simulink model "ele"  (R2023a)
settings: Solver=VariableStepAuto  StartTime=0.0  StopTime=20  RelTol=1e-3
values from neighbouring files (symbols this model uses):
  waypointData_front = [-1.88818518125 -2.2600318378 -2.41179824016 -2.35548053674 -2.22744803538 -2.06210458742 -1.82611832354 -1.58946605338 -1.25340747671 -1.54604493893 -1.70384741821 -1.82785013395 ... (45 elements, 15x3)]    [dat.mat]
  waypointData_hind = [-1.88818518125 -1.55059762067 -1.31714165015 -1.07851127829 -0.915846032516 -0.785511813404 -0.729794322428 -0.881560682034 -1.25340747671 -1.16436080646 -1.21961717711 -1.31374250977 ... (45 elements, 15x3)]    [dat.mat]
undefined symbols (not defined in the file or in its folder): X, Y, Z
libraries: sm_lib x122, nesl_utility x62, robotmaniplib x16, robotcorelib x16
(part 1 of 4)
settings Model: Creator=mkris  LastModifiedBy=mkris

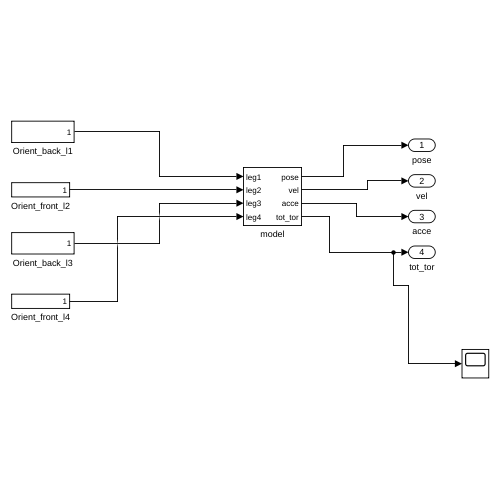
[thumbnail: Simulink's stored preview of the top-level diagram]
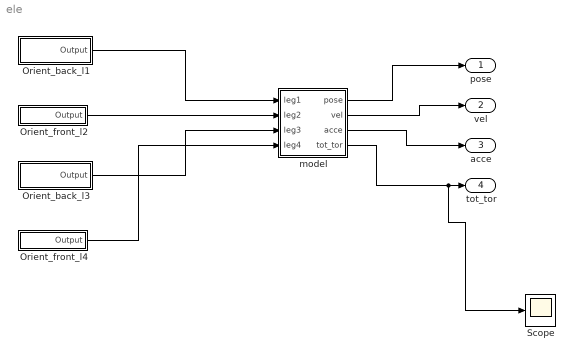
== system ele ==
  Orient_back_l1 : Subsystem
  Orient_back_l3 : Subsystem
  Orient_front_l2 : Subsystem
  Orient_front_l4 : Subsystem
  Scope : Scope
  model : Subsystem
  pose : Outport
  vel : Outport  Port=2
  acce : Outport  Port=3
  tot_tor : Outport  Port=4
  wires:
  model/1(pose) -> pose/1
  model/2(vel) -> vel/1
  model/3(acce) -> acce/1
  model/4(tot_tor) -> Scope/1, tot_tor/1
  Orient_back_l1/1(Output) -> model/1(leg1)
  Orient_front_l2/1(Output) -> model/2(leg2)
  Orient_back_l3/1(Output) -> model/3(leg3)
  Orient_front_l4/1(Output) -> model/4(leg4)

== system ele/Orient_back_l1 ==
  Clock1 : Clock
  If : If  IfExpression=u1 < 5  ElseIfExpressions=u1 < 10,u1 < 15
  Merge : Merge  Inputs=4
  down2 : Subsystem  TreatAsAtomicUnit=on
  down3 : Subsystem  TreatAsAtomicUnit=on
  down4 : Subsystem  TreatAsAtomicUnit=on
  up : Subsystem  TreatAsAtomicUnit=on
  Output : Outport
  wires:
  down4/1(Out1) -> Merge/3
  down3/1(Out1) -> Merge/4
  If/4 -> down4/Action
  If/3 -> down3/Action
  If/2 -> down2/Action
  up/1(Output) -> Merge/1
  Clock1/1 -> If/1, up/1(Input), down2/1(In1), down3/1(In1), down4/1(In1)
  down2/1(Out1) -> Merge/2
  If/1 -> up/Action
  Merge/1 -> Output/1

== system ele/Orient_back_l3 ==
  Clock1 : Clock
  If : If  IfExpression=u1 < 5  ElseIfExpressions=u1 < 10,u1 < 15
  Merge : Merge  Inputs=4
  down2 : Subsystem  TreatAsAtomicUnit=on
  down3 : Subsystem  TreatAsAtomicUnit=on
  down4 : Subsystem  TreatAsAtomicUnit=on
  up : Subsystem  TreatAsAtomicUnit=on
  Output : Outport
  wires:
  Merge/1 -> Output/1
  If/1 -> down3/Action
  down4/1(Out1) -> Merge/2
  Clock1/1 -> down2/1(In1), up/1(Input), down4/1(In1), down3/1(In1), If/1
  down3/1(Out1) -> Merge/1
  If/2 -> down4/Action
  If/3 -> up/Action
  If/4 -> down2/Action
  up/1(Output) -> Merge/4
  down2/1(Out1) -> Merge/3

== system ele/Orient_front_l2 ==
  Clock1 : Clock
  If : If  IfExpression=u1 < 5  ElseIfExpressions=u1 < 10,u1 < 15
  Merge : Merge  Inputs=4
  down2 : Subsystem  TreatAsAtomicUnit=on
  down3 : Subsystem  TreatAsAtomicUnit=on
  down4 : Subsystem  TreatAsAtomicUnit=on
  up : Subsystem  TreatAsAtomicUnit=on
  Output : Outport
  wires:
  If/1 -> down4/Action
  up/1(Output) -> Merge/2
  Clock1/1 -> down2/1(In1), down3/1(In1), up/1(Input), down4/1(In1), If/1
  down4/1(Out1) -> Merge/1
  If/2 -> up/Action
  If/3 -> down2/Action
  If/4 -> down3/Action
  down2/1(Out1) -> Merge/4
  down3/1(Out1) -> Merge/3
  Merge/1 -> Output/1

== system ele/Orient_front_l4 ==
  Clock1 : Clock
  If : If  IfExpression=u1 < 5  ElseIfExpressions=u1 < 10,u1 < 15
  Merge : Merge  Inputs=4
  down2 : Subsystem  TreatAsAtomicUnit=on
  down3 : Subsystem  TreatAsAtomicUnit=on
  down4 : Subsystem  TreatAsAtomicUnit=on
  up : Subsystem  TreatAsAtomicUnit=on
  Output : Outport
  wires:
  Merge/1 -> Output/1
  up/1(Output) -> Merge/3
  down4/1(Out1) -> Merge/4
  If/4 -> up/Action
  If/3 -> down4/Action
  If/2 -> down3/Action
  down2/1(Out1) -> Merge/1
  Clock1/1 -> down3/1(In1), down2/1(In1), If/1, down4/1(In1), up/1(Input)
  down3/1(Out1) -> Merge/2
  If/1 -> down2/Action

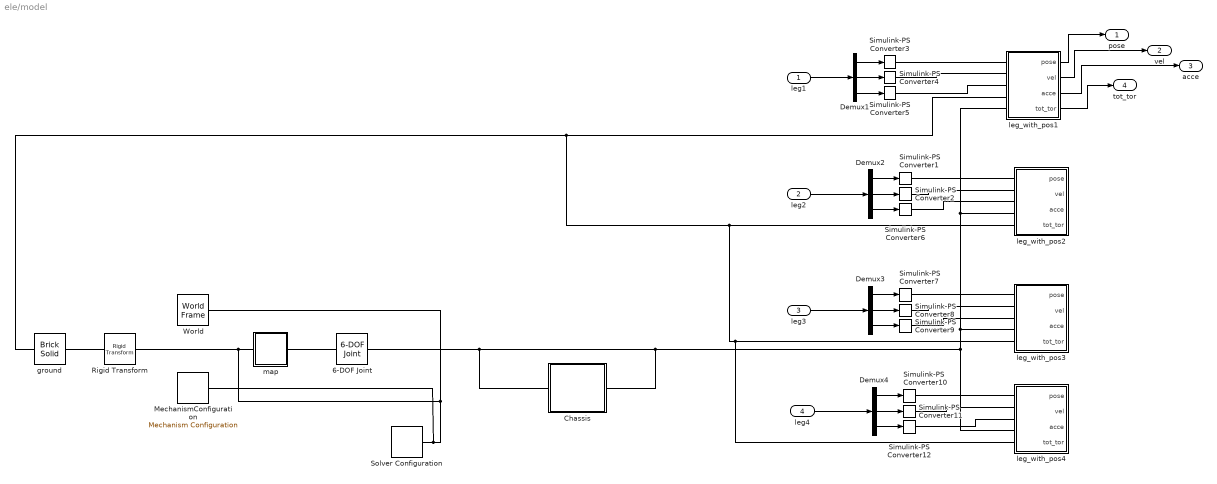
== system ele/model ==
  leg1 : Inport
  leg2 : Inport  Port=2
  leg3 : Inport  Port=3
  leg4 : Inport  Port=4
  6-DOF Joint : sm_lib/Joints/6-DOF Joint  JointMode=Normal  SenseConstraintForce=off  SenseConstraintForceX=off  SenseConstraintForceY=off  SenseConstraintForceZ=off  SenseConstraintTorque=off  SenseConstraintTorqueX=off  SenseConstraintTorqueY=off  SenseConstraintTorqueZ=off  SenseTotalForce=off  SenseTotalForceX=off  SenseTotalForceY=off  SenseTotalForceZ=off  SenseTotalTorque=off  SenseTotalTorqueX=off  SenseTotalTorqueY=off  SenseTotalTorqueZ=off  CompositeWrenchDir=FollowerOnBase  CompositeWrenchFrame=BaseFrame  PxEquilibriumPosition=0  PxEquilibriumPositionUnits=m  PxSpringStiffness=0  PxSpringStiffnessUnits=N/m  PxDampingCoefficient=0  PxDampingCoefficientUnits=N/(m/s)  PxTorqueActuationMode=NoTorque  PxMotionActuationMode=ComputedMotion  PxSensePosition=off  PxSenseVelocity=off  PxSenseAcceleration=off  PxSenseTorqueForce=off  PxSenseLowerLimitTorqueForce=off  PxSenseUpperLimitTorqueForce=off  PxLowerLimitSpecify=off  PxLowerLimitBound=-1  PxLowerLimitBoundUnits=m  PxLowerLimitStiffness=1e6  PxLowerLimitStiffnessUnits=N/m  PxLowerLimitDamping=1e3  PxLowerLimitDampingUnits=N/(m/s)  PxLowerLimitTransitionRegionWidth=1e-4  PxLowerLimitTransitionRegionWidthUnits=m  PxUpperLimitSpecify=off  PxUpperLimitBound=1  PxUpperLimitBoundUnits=m  PxUpperLimitStiffness=1e6  PxUpperLimitStiffnessUnits=N/m  PxUpperLimitDamping=1e3  PxUpperLimitDampingUnits=N/(m/s)  PxUpperLimitTransitionRegionWidth=1e-4  PxUpperLimitTransitionRegionWidthUnits=m  PxPositionTargetSpecify=off  PxPositionTargetPriority=High  PxPositionTargetValue=0  PxPositionTargetValueUnits=m  PxVelocityTargetSpecify=off  PxVelocityTargetPriority=High  PxVelocityTargetValue=0  PxVelocityTargetValueUnits=m/s  PyEquilibriumPosition=0  PyEquilibriumPositionUnits=m  PySpringStiffness=0  PySpringStiffnessUnits=N/m  PyDampingCoefficient=0  PyDampingCoefficientUnits=N/(m/s)  PyTorqueActuationMode=NoTorque  PyMotionActuationMode=ComputedMotion  PySensePosition=off  PySenseVelocity=off  PySenseAcceleration=off  PySenseTorqueForce=off  PySenseLowerLimitTorqueForce=off  PySenseUpperLimitTorqueForce=off  PyLowerLimitSpecify=off  PyLowerLimitBound=-1  PyLowerLimitBoundUnits=m  PyLowerLimitStiffness=1e6  PyLowerLimitStiffnessUnits=N/m  PyLowerLimitDamping=1e3  PyLowerLimitDampingUnits=N/(m/s)  PyLowerLimitTransitionRegionWidth=1e-4  PyLowerLimitTransitionRegionWidthUnits=m  PyUpperLimitSpecify=off  PyUpperLimitBound=1  PyUpperLimitBoundUnits=m  PyUpperLimitStiffness=1e6  PyUpperLimitStiffnessUnits=N/m  PyUpperLimitDamping=1e3  PyUpperLimitDampingUnits=N/(m/s)  PyUpperLimitTransitionRegionWidth=1e-4  PyUpperLimitTransitionRegionWidthUnits=m  PyPositionTargetSpecify=off  PyPositionTargetPriority=High  PyPositionTargetValue=0  PyPositionTargetValueUnits=m  PyVelocityTargetSpecify=off  PyVelocityTargetPriority=High  PyVelocityTargetValue=0  PyVelocityTargetValueUnits=m/s  PzEquilibriumPosition=0  PzEquilibriumPositionUnits=m  PzSpringStiffness=0  PzSpringStiffnessUnits=N/m  PzDampingCoefficient=0  PzDampingCoefficientUnits=N/(m/s)  PzTorqueActuationMode=NoTorque  PzMotionActuationMode=ComputedMotion  PzSensePosition=off  PzSenseVelocity=off  PzSenseAcceleration=off  PzSenseTorqueForce=off  PzSenseLowerLimitTorqueForce=off  PzSenseUpperLimitTorqueForce=off  PzLowerLimitSpecify=off  PzLowerLimitBound=-1  PzLowerLimitBoundUnits=m  PzLowerLimitStiffness=1e6  PzLowerLimitStiffnessUnits=N/m  PzLowerLimitDamping=1e3  PzLowerLimitDampingUnits=N/(m/s)  PzLowerLimitTransitionRegionWidth=1e-4  PzLowerLimitTransitionRegionWidthUnits=m  PzUpperLimitSpecify=off  PzUpperLimitBound=1  PzUpperLimitBoundUnits=m  PzUpperLimitStiffness=1e6  PzUpperLimitStiffnessUnits=N/m  PzUpperLimitDamping=1e3  PzUpperLimitDampingUnits=N/(m/s)  PzUpperLimitTransitionRegionWidth=1e-4  PzUpperLimitTransitionRegionWidthUnits=m  PzPositionTargetSpecify=off  PzPositionTargetPriority=High  PzPositionTargetValue=0  PzPositionTargetValueUnits=m  PzVelocityTargetSpecify=off  PzVelocityTargetPriority=High  PzVelocityTargetValue=0  PzVelocityTargetValueUnits=m/s  SphEqPosRotationMethod=None  SphEqPosRotationAngleUnits=deg  SphEqPosRotationStandardAxis=+Z  SphEqPosRotationAngle=0.0  SphEqPosRotationArbitraryAxis=[0 0 1]  SphEqPosFollAlignAxisA=+X  SphEqPosBaseAlignAxisA=+Y  SphEqPosFollAlignAxisB=+Y  SphEqPosBaseAlignAxisB=+Z  SphEqPosRotationSequenceAxes=FollowerAxes  SphEqPosRotationSequence=XYX  SphEqPosRotationSequenceAngles=[0 0 0]  SphEqPosRotationSequenceAnglesUnits=deg  SphEqPosRotationMatrix=[1 0 0; 0 1 0; 0 0 1]  SphEqPosQuaternion=[1 0 0 0]  SphSpringStiffness=0  SphSpringStiffnessUnits=N*m/deg  SphDampingCoefficient=0  SphDampingCoefficientUnits=N*m/(deg/s)  SphActuateTorqueX=off  SphActuateTorqueY=off  SphActuateTorqueZ=off  SphActuateTorque=off  SphTorqueActuationMode=NoTorque  SphMotionActuationMode=ComputedMotion  SphActuationFrame=BaseFrame  SphSensePosition=off  SphSenseVelocityX=off  SphSenseVelocityY=off  SphSenseVelocityZ=off  SphSenseVelocity=off  SphSenseAccelerationX=off  SphSenseAccelerationY=off  SphSenseAccelerationZ=off  SphSenseAcceleration=off  SphSenseTorqueX=off  SphSenseTorqueY=off  SphSenseTorqueZ=off  SphSenseTorqueForce=off  SphSenseLowerLimitTorqueMag=off  SphSenseUpperLimitTorqueMag=off  SphSensingFrame=BaseFrame  SphLowerLimitSpecify=off  SphLowerLimitBound=15  SphLowerLimitBoundUnits=deg  SphLowerLimitStiffness=1e4  SphLowerLimitStiffnessUnits=N*m/deg  SphLowerLimitDamping=10  SphLowerLimitDampingUnits=N*m/(deg/s)  SphLowerLimitTransitionRegionWidth=0.1  SphLowerLimitTransitionRegionWidthUnits=deg  SphUpperLimitSpecify=off  SphUpperLimitBound=45  SphUpperLimitBoundUnits=deg  SphUpperLimitStiffness=1e4  SphUpperLimitStiffnessUnits=N*m/deg  SphUpperLimitDamping=10  SphUpperLimitDampingUnits=N*m/(deg/s)  SphUpperLimitTransitionRegionWidth=0.1  SphUpperLimitTransitionRegionWidthUnits=deg  SphPositionTargetRotationMethod=None  SphPositionTargetRotationAngleUnits=deg  SphPositionTargetRotationStandardAxis=+Z  SphPositionTargetRotationAngle=0.0  SphPositionTargetRotationArbitraryAxis=[0 0 1]  SphPositionTargetFollAlignAxisA=+X  SphPositionTargetBaseAlignAxisA=+Y  SphPositionTargetFollAlignAxisB=+Y  SphPositionTargetBaseAlignAxisB=+Z  SphPositionTargetRotationSequenceAxes=FollowerAxes  SphPositionTargetRotationSequence=XYX  SphPositionTargetRotationSequenceAngles=[0 0 0]  SphPositionTargetRotationSequenceAnglesUnits=deg  SphPositionTargetRotationMatrix=[1 0 0; 0 1 0; 0 0 1]  SphPositionTargetQuaternion=[1 0 0 0]  SphPositionTargetSpecify=off  SphPositionTargetPriority=High  SphVelocityTargetValue=[0 0 0]  SphVelocityTargetValueUnits=deg/s  SphVelocityTargetSpecify=off  SphVelocityTargetPriority=High  SphVelocityTargetInFollowerFrame=on
  Chassis : Subsystem
  Demux{1..4} (4 alike) : Demux  Outputs=3
  MechanismConfiguration : sm_lib/Utilities/Mechanism Configuration  UniformGravity=Constant  GravityVector=[0 0 -9.80665]  GravityVectorUnits=m/s^2  LinearizationDelta=0.001  JointModeTransitionNonlinearIterations=2
  Rigid Transform : sm_lib/Frames and Transforms/Rigid Transform  TranslationMethod=Cartesian  TranslationStandardOffset=0  TranslationStandardOffsetUnits=m  TranslationStandardAxis=+Z  TranslationCartesianOffset=[0 0 12.5]  TranslationCartesianOffsetUnits=m  TranslationROffset=0  TranslationROffsetUnits=m  TranslationZOffset=0  TranslationZOffsetUnits=m  TranslationThetaOffset=0  TranslationThetaOffsetUnits=deg  RotationMethod=None  RotationAngleUnits=deg  RotationStandardAxis=+Z  RotationAngle=0.0  RotationArbitraryAxis=[0 0 1]  FollAlignAxisA=+X  BaseAlignAxisA=+Y  FollAlignAxisB=+Y  BaseAlignAxisB=+Z  RotationSequenceAxes=FollowerAxes  RotationSequence=XYX  RotationSequenceAngles=[0 0 0]  RotationSequenceAnglesUnits=deg  RotationMatrix=[1 0 0; 0 1 0; 0 0 1]  Quaternion=[1 0 0 0]
  Simulink-PS Converter{1..12} (12 alike) : nesl_utility/Simulink-PS Converter  PhysicalDomain=network_engine_domain  SubClassName=ps_input  LeftPortType=input  RightPortType=output  PseudoPeriodic=off  Frequencies=[]  NoiseDistribution=none  NoiseParameters=[]  Unit=1  AffineConversion=off  FilteringAndDerivatives=filter  SimscapeFilterOrder=2  InputFilterTimeConstant=0.001  UdotUserProvided=0
  Solver Configuration : nesl_utility/Solver Configuration  PhysicalDomain=network_engine_domain  SubClassName=solver  LeftPortType=input  RightPortType=generic  Tones=[]  Harmonics=[]  SimulateNoise=off  Profile=off  UseLocalSampling=off  EnableSwitchedLinearOptims=on  FrequencyDomain=off  UseCCode=off  RelTol=0.001  AbsTol=0.001  MinStep=1e-09  ToWorkspace=off  RevertToSquareIcSolve=off  NumHomotopyIterations=100  PhasorMode=off  PhasorModeNumHarmonics=1  ConsistencySolver=NEWTON_XTOL_AFTER_FTOL  IndexReductionMethod=DerivativeReplacement  DoDC=off  ResidualTolerance=1e-09  ConsistencyTolSource=GLOBAL  ConsistencyAbsTol=0.001  ConsistencyRelTol=0.001  ConsistencyTolFactor=0.001  UseLocalSolver=off  LocalSolverChoice=NE_BACKWARD_EULER_ADVANCER  ResolveIndetEquations=on  FunctionEvalNumThread=1  LocalSolverSampleTime=0.001  DoFixedCost=off  MaxNonlinIter=3  MaxModeIter=2  ComputeImpulses=off  ImpulseIterations=2  LinearAlgebra=auto  LinearAlgebraNumThread=0  EquationFormulation=NE_TIME_EF  DelaysMemoryBudget=1024  AutomaticFiltering=on  FilteringTimeConstant=0.001  PartitionStorageMethod=AS_NEEDED  PartitionMemoryBudget=1024  PartitionMethod=ROBUST
  World : sm_lib/Frames and Transforms/World Frame
  ground : sm_lib/Body Elements/Brick Solid  GraphicAmbientColor=[0.15 0.15 0.15 1.0]  BasedOnType=Density  BrickDimensions=[100 100 2]  BrickDimensionsUnits=m  CenterOfMass=[0 0 0]  CenterOfMassUnits=m  GraphicDiffuseColor=[0.5 0.5 0.5]  Density=1000  DensityUnits=kg/m^3  DoExposeReferenceFrame=on  GraphicEmissiveColor=[0.0 0.0 0.0 1.0]  ExportEntireGeometry=on  SerializedFrames=<Frames/>  MarkerShape=Sphere  MarkerSize=10  GraphicType=FromGeometry  InertiaType=Custom  Mass=1  MassUnits=kg  MomentsOfInertia=[0 0 0]  MomentsOfInertiaUnits=kg*m^2  GraphicOpacity=1.0  ProductsOfInertia=[0 0 0]  ProductsOfInertiaUnits=kg*m^2  GraphicShininess=75  GraphicSpecularColor=[0.5 0.5 0.5 1.0]  GraphicVisPropType=SimpleVisualProperties
  leg_with_pos1 : Subsystem
  leg_with_pos2 : Subsystem
  leg_with_pos3 : Subsystem
  leg_with_pos4 : Subsystem
  map : Subsystem
  pose : Outport
  vel : Outport  Port=2
  acce : Outport  Port=3
  tot_tor : Outport  Port=4
  wires:
  leg_with_pos1/1(pose) -> pose/1
  leg_with_pos1/2(vel) -> vel/1
  leg_with_pos1/3(acce) -> acce/1
  leg_with_pos1/4(tot_tor) -> tot_tor/1
  leg1/1 -> Demux1/1
  Demux1/2 -> Simulink-PS Converter4/1
  Demux1/1 -> Simulink-PS Converter3/1
  Demux1/3 -> Simulink-PS Converter5/1
  leg3/1 -> Demux3/1
  Demux3/2 -> Simulink-PS Converter8/1
  Demux3/1 -> Simulink-PS Converter7/1
  Demux3/3 -> Simulink-PS Converter9/1
  Demux2/3 -> Simulink-PS Converter6/1
  Demux2/1 -> Simulink-PS Converter1/1
  Demux2/2 -> Simulink-PS Converter2/1
  leg2/1 -> Demux2/1
  leg4/1 -> Demux4/1
  Demux4/2 -> Simulink-PS Converter11/1
  Demux4/1 -> Simulink-PS Converter10/1
  Demux4/3 -> Simulink-PS Converter12/1
  connections:
  ground/RConn1 -- Rigid Transform/LConn1
  6-DOF Joint/LConn1 -- map/RConn1
  6-DOF Joint/RConn1 -- Chassis/LConn1 -- Chassis/RConn1 -- leg_with_pos4/LConn4 -- leg_with_pos3/LConn4 -- leg_with_pos2/LConn4 -- leg_with_pos1/LConn5
  Simulink-PS Converter4/RConn1 -- leg_with_pos1/LConn2
  Simulink-PS Converter3/RConn1 -- leg_with_pos1/LConn1
  Simulink-PS Converter5/RConn1 -- leg_with_pos1/LConn3
  leg_with_pos3/LConn2 -- Simulink-PS Converter8/RConn1
  leg_with_pos3/LConn1 -- Simulink-PS Converter7/RConn1
  leg_with_pos3/LConn3 -- Simulink-PS Converter9/RConn1
  leg_with_pos2/LConn2 -- Simulink-PS Converter2/RConn1
  leg_with_pos2/LConn1 -- Simulink-PS Converter1/RConn1
  leg_with_pos2/LConn3 -- Simulink-PS Converter6/RConn1
  leg_with_pos4/LConn2 -- Simulink-PS Converter11/RConn1
  leg_with_pos4/LConn1 -- Simulink-PS Converter10/RConn1
  leg_with_pos4/LConn3 -- Simulink-PS Converter12/RConn1
  MechanismConfiguration/RConn1 -- World/RConn1 -- Rigid Transform/RConn1 -- map/LConn1 -- Solver Configuration/RConn1
  ground/LConn1 -- leg_with_pos4/LConn5 -- leg_with_pos3/LConn5 -- leg_with_pos2/LConn5 -- leg_with_pos1/LConn4

== system ele/Orient_back_l1/down2 ==
  In1 : Inport
  Action Port : ActionPort  ActionPortLabel=elseif(u1 < 10)
  Joint Space Motion Model1 : robotmaniplib/Joint Space Motion Model  RigidBodyTree=ele  MotionType=Independent Joint Motion  ProportionalGain=100  DerivativeGain=10  ErrorDynamicsSpecification=Damping Ratio / Natural Frequency  DampingRatio=1  NaturalFrequency=10  SettlingTime=0.59  Overshoot=0  ShowExternalForcePort=off  InitConfig=waypointData_hind(9,:)  InitJointVel=0  SimulateUsing=Interpreted execution
  Polynomial Trajectory1 : robotcorelib/Polynomial Trajectory  WaypointSource=Internal  Waypoints=waypointData_hind(9:11,:)'  TimePoints=linspace(5,10,3)  TimeInterval=[ 1, 4 ]  Method=Cubic Polynomial  ParameterSource=Internal  VelocityBoundaryCondition=zeros( 3, 3)  AccelerationBoundaryCondition=zeros( 3, 50)  SimulateUsing=Code generation
  Scope : Scope
  Scope3 : Scope
  Terminator2 : Terminator
  Terminator3 : Terminator
  Out1 : Outport
  wires:
  Joint Space Motion Model1/1 -> Scope/1, Out1/1
  Joint Space Motion Model1/3 -> Terminator3/1
  In1/1 -> Polynomial Trajectory1/1
  Polynomial Trajectory1/2 -> Joint Space Motion Model1/2
  Polynomial Trajectory1/3 -> Joint Space Motion Model1/3
  Polynomial Trajectory1/1 -> Joint Space Motion Model1/1, Scope3/1
  Joint Space Motion Model1/2 -> Terminator2/1

== system ele/Orient_back_l1/down3 ==
  In1 : Inport
  Action Port : ActionPort  ActionPortLabel=elseif(u1 < 15)
  Joint Space Motion Model1 : robotmaniplib/Joint Space Motion Model  RigidBodyTree=ele  MotionType=Independent Joint Motion  ProportionalGain=100  DerivativeGain=10  ErrorDynamicsSpecification=Damping Ratio / Natural Frequency  DampingRatio=1  NaturalFrequency=10  SettlingTime=0.59  Overshoot=0  ShowExternalForcePort=off  InitConfig=waypointData_hind(11,:)  InitJointVel=0  SimulateUsing=Interpreted execution
  Polynomial Trajectory1 : robotcorelib/Polynomial Trajectory  WaypointSource=Internal  Waypoints=waypointData_hind(11:13,:)'  TimePoints=linspace(10,15,3)  TimeInterval=[ 1, 4 ]  Method=Cubic Polynomial  ParameterSource=Internal  VelocityBoundaryCondition=zeros( 3, 3)  AccelerationBoundaryCondition=zeros( 3, 50)  SimulateUsing=Code generation
  Scope : Scope
  Scope3 : Scope
  Terminator2 : Terminator
  Terminator3 : Terminator
  Out1 : Outport
  wires:
  Joint Space Motion Model1/2 -> Terminator2/1
  Polynomial Trajectory1/1 -> Scope3/1, Joint Space Motion Model1/1
  Polynomial Trajectory1/3 -> Joint Space Motion Model1/3
  Polynomial Trajectory1/2 -> Joint Space Motion Model1/2
  In1/1 -> Polynomial Trajectory1/1
  Joint Space Motion Model1/3 -> Terminator3/1
  Joint Space Motion Model1/1 -> Out1/1, Scope/1

== system ele/Orient_back_l1/down4 ==
  In1 : Inport
  Action Port : ActionPort  ActionPortLabel=else
  Joint Space Motion Model1 : robotmaniplib/Joint Space Motion Model  RigidBodyTree=ele  MotionType=Independent Joint Motion  ProportionalGain=100  DerivativeGain=10  ErrorDynamicsSpecification=Damping Ratio / Natural Frequency  DampingRatio=1  NaturalFrequency=10  SettlingTime=0.59  Overshoot=0  ShowExternalForcePort=off  InitConfig=waypointData_hind(13,:)  InitJointVel=0  SimulateUsing=Interpreted execution
  Polynomial Trajectory1 : robotcorelib/Polynomial Trajectory  WaypointSource=Internal  Waypoints=waypointData_hind(13:15,:)'  TimePoints=linspace(15,20,3)  TimeInterval=[ 1, 4 ]  Method=Cubic Polynomial  ParameterSource=Internal  VelocityBoundaryCondition=zeros( 3, 3)  AccelerationBoundaryCondition=zeros( 3, 50)  SimulateUsing=Code generation
  Scope : Scope
  Scope3 : Scope
  Terminator2 : Terminator
  Terminator3 : Terminator
  Out1 : Outport
  wires:
  Joint Space Motion Model1/1 -> Scope/1, Out1/1
  Joint Space Motion Model1/3 -> Terminator3/1
  In1/1 -> Polynomial Trajectory1/1
  Polynomial Trajectory1/2 -> Joint Space Motion Model1/2
  Polynomial Trajectory1/3 -> Joint Space Motion Model1/3
  Polynomial Trajectory1/1 -> Joint Space Motion Model1/1, Scope3/1
  Joint Space Motion Model1/2 -> Terminator2/1

== system ele/Orient_back_l1/up ==
  Input : Inport
  Action Port : ActionPort  ActionPortLabel=if(u1 < 5)
  Joint Space Motion Model : robotmaniplib/Joint Space Motion Model  RigidBodyTree=ele  MotionType=Independent Joint Motion  ProportionalGain=100  DerivativeGain=10  ErrorDynamicsSpecification=Damping Ratio / Natural Frequency  DampingRatio=1  NaturalFrequency=10  SettlingTime=0.59  Overshoot=0  ShowExternalForcePort=off  InitConfig=waypointData_hind(1,:)  InitJointVel=0  SimulateUsing=Interpreted execution
  Polynomial Trajectory : robotcorelib/Polynomial Trajectory  WaypointSource=Internal  Waypoints=waypointData_hind(1:9,:)'  TimePoints=linspace(0,5,9)  TimeInterval=[ 1, 4 ]  Method=Cubic Polynomial  ParameterSource=Internal  VelocityBoundaryCondition=zeros( 3, 9)  AccelerationBoundaryCondition=zeros( 3, 50)  SimulateUsing=Code generation
  Scope1 : Scope
  Scope2 : Scope
  Terminator : Terminator
  Terminator1 : Terminator
  Output : Outport
  wires:
  Input/1 -> Polynomial Trajectory/1
  Polynomial Trajectory/1 -> Scope1/1, Joint Space Motion Model/1
  Polynomial Trajectory/2 -> Joint Space Motion Model/2
  Joint Space Motion Model/1 -> Scope2/1, Output/1
  Joint Space Motion Model/3 -> Terminator1/1
  Polynomial Trajectory/3 -> Joint Space Motion Model/3
  Joint Space Motion Model/2 -> Terminator/1

== system ele/Orient_back_l3/down2 ==
  In1 : Inport
  Action Port : ActionPort  ActionPortLabel=else
  Joint Space Motion Model1 : robotmaniplib/Joint Space Motion Model  RigidBodyTree=ele  MotionType=Independent Joint Motion  ProportionalGain=100  DerivativeGain=10  ErrorDynamicsSpecification=Damping Ratio / Natural Frequency  DampingRatio=1  NaturalFrequency=10  SettlingTime=0.59  Overshoot=0  ShowExternalForcePort=off  InitConfig=waypointData_hind(9,:)  InitJointVel=0  SimulateUsing=Interpreted execution
  Polynomial Trajectory1 : robotcorelib/Polynomial Trajectory  WaypointSource=Internal  Waypoints=waypointData_hind(9:11,:)'  TimePoints=linspace(15,20,3)  TimeInterval=[ 1, 4 ]  Method=Cubic Polynomial  ParameterSource=Internal  VelocityBoundaryCondition=zeros( 3, 3)  AccelerationBoundaryCondition=zeros( 3, 50)  SimulateUsing=Code generation
  Scope : Scope
  Scope3 : Scope
  Terminator2 : Terminator
  Terminator3 : Terminator
  Out1 : Outport
  wires:
  Joint Space Motion Model1/2 -> Terminator2/1
  Polynomial Trajectory1/1 -> Scope3/1, Joint Space Motion Model1/1
  Polynomial Trajectory1/3 -> Joint Space Motion Model1/3
  Polynomial Trajectory1/2 -> Joint Space Motion Model1/2
  In1/1 -> Polynomial Trajectory1/1
  Joint Space Motion Model1/3 -> Terminator3/1
  Joint Space Motion Model1/1 -> Out1/1, Scope/1

== system ele/Orient_back_l3/down3 ==
  In1 : Inport
  Action Port : ActionPort  ActionPortLabel=if(u1 < 5)
  Joint Space Motion Model1 : robotmaniplib/Joint Space Motion Model  RigidBodyTree=ele  MotionType=Independent Joint Motion  ProportionalGain=100  DerivativeGain=10  ErrorDynamicsSpecification=Damping Ratio / Natural Frequency  DampingRatio=1  NaturalFrequency=10  SettlingTime=0.59  Overshoot=0  ShowExternalForcePort=off  InitConfig=waypointData_hind(11,:)  InitJointVel=0  SimulateUsing=Interpreted execution
  Polynomial Trajectory1 : robotcorelib/Polynomial Trajectory  WaypointSource=Internal  Waypoints=waypointData_hind(11:13,:)'  TimePoints=linspace(0,5,3)  TimeInterval=[ 1, 4 ]  Method=Cubic Polynomial  ParameterSource=Internal  VelocityBoundaryCondition=zeros( 3, 3)  AccelerationBoundaryCondition=zeros( 3, 50)  SimulateUsing=Code generation
  Scope : Scope
  Scope3 : Scope
  Terminator2 : Terminator
  Terminator3 : Terminator
  Out1 : Outport
  wires:
  Joint Space Motion Model1/1 -> Scope/1, Out1/1
  Joint Space Motion Model1/3 -> Terminator3/1
  In1/1 -> Polynomial Trajectory1/1
  Polynomial Trajectory1/2 -> Joint Space Motion Model1/2
  Polynomial Trajectory1/3 -> Joint Space Motion Model1/3
  Polynomial Trajectory1/1 -> Joint Space Motion Model1/1, Scope3/1
  Joint Space Motion Model1/2 -> Terminator2/1

== system ele/Orient_back_l3/down4 ==
  In1 : Inport
  Action Port : ActionPort  ActionPortLabel=elseif(u1 < 10)
  Joint Space Motion Model1 : robotmaniplib/Joint Space Motion Model  RigidBodyTree=ele  MotionType=Independent Joint Motion  ProportionalGain=100  DerivativeGain=10  ErrorDynamicsSpecification=Damping Ratio / Natural Frequency  DampingRatio=1  NaturalFrequency=10  SettlingTime=0.59  Overshoot=0  ShowExternalForcePort=off  InitConfig=waypointData_hind(13,:)  InitJointVel=0  SimulateUsing=Interpreted execution
  Polynomial Trajectory1 : robotcorelib/Polynomial Trajectory  WaypointSource=Internal  Waypoints=waypointData_hind(13:15,:)'  TimePoints=linspace(5,10,3)  TimeInterval=[ 1, 4 ]  Method=Cubic Polynomial  ParameterSource=Internal  VelocityBoundaryCondition=zeros( 3, 3)  AccelerationBoundaryCondition=zeros( 3, 50)  SimulateUsing=Code generation
  Scope : Scope
  Scope3 : Scope
  Terminator2 : Terminator
  Terminator3 : Terminator
  Out1 : Outport
  wires:
  Joint Space Motion Model1/2 -> Terminator2/1
  Polynomial Trajectory1/1 -> Scope3/1, Joint Space Motion Model1/1
  Polynomial Trajectory1/3 -> Joint Space Motion Model1/3
  Polynomial Trajectory1/2 -> Joint Space Motion Model1/2
  In1/1 -> Polynomial Trajectory1/1
  Joint Space Motion Model1/3 -> Terminator3/1
  Joint Space Motion Model1/1 -> Out1/1, Scope/1

== system ele/Orient_back_l3/up ==
  Input : Inport
  Action Port : ActionPort  ActionPortLabel=elseif(u1 < 15)
  Joint Space Motion Model : robotmaniplib/Joint Space Motion Model  RigidBodyTree=ele  MotionType=Independent Joint Motion  ProportionalGain=100  DerivativeGain=10  ErrorDynamicsSpecification=Damping Ratio / Natural Frequency  DampingRatio=1  NaturalFrequency=10  SettlingTime=0.59  Overshoot=0  ShowExternalForcePort=off  InitConfig=waypointData_hind(1,:)  InitJointVel=0  SimulateUsing=Interpreted execution
  Polynomial Trajectory : robotcorelib/Polynomial Trajectory  WaypointSource=Internal  Waypoints=waypointData_hind(1:9,:)'  TimePoints=linspace(10,15,9)  TimeInterval=[ 1, 4 ]  Method=Cubic Polynomial  ParameterSource=Internal  VelocityBoundaryCondition=zeros( 3, 9)  AccelerationBoundaryCondition=zeros( 3, 50)  SimulateUsing=Code generation
  Scope1 : Scope
  Scope2 : Scope
  Terminator : Terminator
  Terminator1 : Terminator
  Output : Outport
  wires:
  Joint Space Motion Model/2 -> Terminator/1
  Polynomial Trajectory/3 -> Joint Space Motion Model/3
  Joint Space Motion Model/3 -> Terminator1/1
  Joint Space Motion Model/1 -> Output/1, Scope2/1
  Polynomial Trajectory/2 -> Joint Space Motion Model/2
  Polynomial Trajectory/1 -> Joint Space Motion Model/1, Scope1/1
  Input/1 -> Polynomial Trajectory/1

== system ele/Orient_front_l2/down2 ==
  In1 : Inport
  Action Port : ActionPort  ActionPortLabel=elseif(u1 < 15)
  Joint Space Motion Model1 : robotmaniplib/Joint Space Motion Model  RigidBodyTree=ele  MotionType=Independent Joint Motion  ProportionalGain=100  DerivativeGain=10  ErrorDynamicsSpecification=Damping Ratio / Natural Frequency  DampingRatio=1  NaturalFrequency=10  SettlingTime=0.59  Overshoot=0  ShowExternalForcePort=off  InitConfig=waypointData_front(9,:)  InitJointVel=0  SimulateUsing=Interpreted execution
  Polynomial Trajectory1 : robotcorelib/Polynomial Trajectory  WaypointSource=Internal  Waypoints=waypointData_front(9:11,:)'  TimePoints=linspace(10,15,3)  TimeInterval=[ 1, 4 ]  Method=Cubic Polynomial  ParameterSource=Internal  VelocityBoundaryCondition=zeros( 3, 3)  AccelerationBoundaryCondition=zeros( 3, 50)  SimulateUsing=Code generation
  Scope : Scope
  Scope3 : Scope
  Terminator2 : Terminator
  Terminator3 : Terminator
  Out1 : Outport
  wires:
  Joint Space Motion Model1/2 -> Terminator2/1
  Polynomial Trajectory1/1 -> Scope3/1, Joint Space Motion Model1/1
  Polynomial Trajectory1/3 -> Joint Space Motion Model1/3
  Polynomial Trajectory1/2 -> Joint Space Motion Model1/2
  In1/1 -> Polynomial Trajectory1/1
  Joint Space Motion Model1/3 -> Terminator3/1
  Joint Space Motion Model1/1 -> Out1/1, Scope/1

== system ele/Orient_front_l2/down3 ==
  In1 : Inport
  Action Port : ActionPort  ActionPortLabel=else
  Joint Space Motion Model1 : robotmaniplib/Joint Space Motion Model  RigidBodyTree=ele  MotionType=Independent Joint Motion  ProportionalGain=100  DerivativeGain=10  ErrorDynamicsSpecification=Damping Ratio / Natural Frequency  DampingRatio=1  NaturalFrequency=10  SettlingTime=0.59  Overshoot=0  ShowExternalForcePort=off  InitConfig=waypointData_front(11,:)  InitJointVel=0  SimulateUsing=Interpreted execution
  Polynomial Trajectory1 : robotcorelib/Polynomial Trajectory  WaypointSource=Internal  Waypoints=waypointData_front(11:13,:)'  TimePoints=linspace(15,20,3)  TimeInterval=[ 1, 4 ]  Method=Cubic Polynomial  ParameterSource=Internal  VelocityBoundaryCondition=zeros( 3, 3)  AccelerationBoundaryCondition=zeros( 3, 50)  SimulateUsing=Code generation
  Scope : Scope
  Scope3 : Scope
  Terminator2 : Terminator
  Terminator3 : Terminator
  Out1 : Outport
  wires:
  Joint Space Motion Model1/1 -> Scope/1, Out1/1
  Joint Space Motion Model1/3 -> Terminator3/1
  In1/1 -> Polynomial Trajectory1/1
  Polynomial Trajectory1/2 -> Joint Space Motion Model1/2
  Polynomial Trajectory1/3 -> Joint Space Motion Model1/3
  Polynomial Trajectory1/1 -> Joint Space Motion Model1/1, Scope3/1
  Joint Space Motion Model1/2 -> Terminator2/1

== system ele/Orient_front_l2/down4 ==
  In1 : Inport
  Action Port : ActionPort  ActionPortLabel=if(u1 < 5)
  Joint Space Motion Model1 : robotmaniplib/Joint Space Motion Model  RigidBodyTree=ele  MotionType=Independent Joint Motion  ProportionalGain=100  DerivativeGain=10  ErrorDynamicsSpecification=Damping Ratio / Natural Frequency  DampingRatio=1  NaturalFrequency=10  SettlingTime=0.59  Overshoot=0  ShowExternalForcePort=off  InitConfig=waypointData_front(13,:)  InitJointVel=0  SimulateUsing=Interpreted execution
  Polynomial Trajectory1 : robotcorelib/Polynomial Trajectory  WaypointSource=Internal  Waypoints=waypointData_front(13:15,:)'  TimePoints=linspace(0,5,3)  TimeInterval=[ 1, 4 ]  Method=Cubic Polynomial  ParameterSource=Internal  VelocityBoundaryCondition=zeros( 3, 3)  AccelerationBoundaryCondition=zeros( 3, 50)  SimulateUsing=Code generation
  Scope : Scope
  Scope3 : Scope
  Terminator2 : Terminator
  Terminator3 : Terminator
  Out1 : Outport
  wires:
  Joint Space Motion Model1/2 -> Terminator2/1
  Polynomial Trajectory1/1 -> Scope3/1, Joint Space Motion Model1/1
  Polynomial Trajectory1/3 -> Joint Space Motion Model1/3
  Polynomial Trajectory1/2 -> Joint Space Motion Model1/2
  In1/1 -> Polynomial Trajectory1/1
  Joint Space Motion Model1/3 -> Terminator3/1
  Joint Space Motion Model1/1 -> Out1/1, Scope/1

== system ele/Orient_front_l2/up ==
  Input : Inport
  Action Port : ActionPort  ActionPortLabel=elseif(u1 < 10)
  Joint Space Motion Model : robotmaniplib/Joint Space Motion Model  RigidBodyTree=ele  MotionType=Independent Joint Motion  ProportionalGain=100  DerivativeGain=10  ErrorDynamicsSpecification=Damping Ratio / Natural Frequency  DampingRatio=1  NaturalFrequency=10  SettlingTime=0.59  Overshoot=0  ShowExternalForcePort=off  InitConfig=waypointData_front(1,:)  InitJointVel=0  SimulateUsing=Interpreted execution
  Polynomial Trajectory : robotcorelib/Polynomial Trajectory  WaypointSource=Internal  Waypoints=waypointData_front(1:9,:)'  TimePoints=linspace(5,10,9)  TimeInterval=[ 1, 4 ]  Method=Cubic Polynomial  ParameterSource=Internal  VelocityBoundaryCondition=zeros( 3, 9)  AccelerationBoundaryCondition=zeros( 3, 50)  SimulateUsing=Code generation
  Scope1 : Scope
  Scope2 : Scope
  Terminator : Terminator
  Terminator1 : Terminator
  Output : Outport
  wires:
  Joint Space Motion Model/2 -> Terminator/1
  Polynomial Trajectory/3 -> Joint Space Motion Model/3
  Joint Space Motion Model/3 -> Terminator1/1
  Joint Space Motion Model/1 -> Output/1, Scope2/1
  Polynomial Trajectory/2 -> Joint Space Motion Model/2
  Polynomial Trajectory/1 -> Joint Space Motion Model/1, Scope1/1
  Input/1 -> Polynomial Trajectory/1

== system ele/Orient_front_l4/down2 ==
  In1 : Inport
  Action Port : ActionPort  ActionPortLabel=if(u1 < 5)
  Joint Space Motion Model1 : robotmaniplib/Joint Space Motion Model  RigidBodyTree=ele  MotionType=Independent Joint Motion  ProportionalGain=100  DerivativeGain=10  ErrorDynamicsSpecification=Damping Ratio / Natural Frequency  DampingRatio=1  NaturalFrequency=10  SettlingTime=0.59  Overshoot=0  ShowExternalForcePort=off  InitConfig=waypointData_front(9,:)  InitJointVel=0  SimulateUsing=Interpreted execution
  Polynomial Trajectory1 : robotcorelib/Polynomial Trajectory  WaypointSource=Internal  Waypoints=waypointData_front(9:11,:)'  TimePoints=linspace(0,5,3)  TimeInterval=[ 1, 4 ]  Method=Cubic Polynomial  ParameterSource=Internal  VelocityBoundaryCondition=zeros( 3, 3)  AccelerationBoundaryCondition=zeros( 3, 50)  SimulateUsing=Code generation
  Scope : Scope
  Scope3 : Scope
  Terminator2 : Terminator
  Terminator3 : Terminator
  Out1 : Outport
  wires:
  Joint Space Motion Model1/1 -> Scope/1, Out1/1
  Joint Space Motion Model1/3 -> Terminator3/1
  In1/1 -> Polynomial Trajectory1/1
  Polynomial Trajectory1/2 -> Joint Space Motion Model1/2
  Polynomial Trajectory1/3 -> Joint Space Motion Model1/3
  Polynomial Trajectory1/1 -> Joint Space Motion Model1/1, Scope3/1
  Joint Space Motion Model1/2 -> Terminator2/1

== system ele/Orient_front_l4/down3 ==
  In1 : Inport
  Action Port : ActionPort  ActionPortLabel=elseif(u1 < 10)
  Joint Space Motion Model1 : robotmaniplib/Joint Space Motion Model  RigidBodyTree=ele  MotionType=Independent Joint Motion  ProportionalGain=100  DerivativeGain=10  ErrorDynamicsSpecification=Damping Ratio / Natural Frequency  DampingRatio=1  NaturalFrequency=10  SettlingTime=0.59  Overshoot=0  ShowExternalForcePort=off  InitConfig=waypointData_front(11,:)  InitJointVel=0  SimulateUsing=Interpreted execution
  Polynomial Trajectory1 : robotcorelib/Polynomial Trajectory  WaypointSource=Internal  Waypoints=waypointData_front(11:13,:)'  TimePoints=linspace(5,10,3)  TimeInterval=[ 1, 4 ]  Method=Cubic Polynomial  ParameterSource=Internal  VelocityBoundaryCondition=zeros( 3, 3)  AccelerationBoundaryCondition=zeros( 3, 50)  SimulateUsing=Code generation
  Scope : Scope
  Scope3 : Scope
  Terminator2 : Terminator
  Terminator3 : Terminator
  Out1 : Outport
  wires:
  Joint Space Motion Model1/2 -> Terminator2/1
  Polynomial Trajectory1/1 -> Scope3/1, Joint Space Motion Model1/1
  Polynomial Trajectory1/3 -> Joint Space Motion Model1/3
  Polynomial Trajectory1/2 -> Joint Space Motion Model1/2
  In1/1 -> Polynomial Trajectory1/1
  Joint Space Motion Model1/3 -> Terminator3/1
  Joint Space Motion Model1/1 -> Out1/1, Scope/1

== system ele/Orient_front_l4/down4 ==
  In1 : Inport
  Action Port : ActionPort  ActionPortLabel=elseif(u1 < 15)
  Joint Space Motion Model1 : robotmaniplib/Joint Space Motion Model  RigidBodyTree=ele  MotionType=Independent Joint Motion  ProportionalGain=100  DerivativeGain=10  ErrorDynamicsSpecification=Damping Ratio / Natural Frequency  DampingRatio=1  NaturalFrequency=10  SettlingTime=0.59  Overshoot=0  ShowExternalForcePort=off  InitConfig=waypointData_front(13,:)  InitJointVel=0  SimulateUsing=Interpreted execution
  Polynomial Trajectory1 : robotcorelib/Polynomial Trajectory  WaypointSource=Internal  Waypoints=waypointData_front(13:15,:)'  TimePoints=linspace(10,15,3)  TimeInterval=[ 1, 4 ]  Method=Cubic Polynomial  ParameterSource=Internal  VelocityBoundaryCondition=zeros( 3, 3)  AccelerationBoundaryCondition=zeros( 3, 50)  SimulateUsing=Code generation
  Scope : Scope
  Scope3 : Scope
  Terminator2 : Terminator
  Terminator3 : Terminator
  Out1 : Outport
  wires:
  Joint Space Motion Model1/1 -> Scope/1, Out1/1
  Joint Space Motion Model1/3 -> Terminator3/1
  In1/1 -> Polynomial Trajectory1/1
  Polynomial Trajectory1/2 -> Joint Space Motion Model1/2
  Polynomial Trajectory1/3 -> Joint Space Motion Model1/3
  Polynomial Trajectory1/1 -> Joint Space Motion Model1/1, Scope3/1
  Joint Space Motion Model1/2 -> Terminator2/1

== system ele/Orient_front_l4/up ==
  Input : Inport
  Action Port : ActionPort  ActionPortLabel=else
  Joint Space Motion Model : robotmaniplib/Joint Space Motion Model  RigidBodyTree=ele  MotionType=Independent Joint Motion  ProportionalGain=100  DerivativeGain=10  ErrorDynamicsSpecification=Damping Ratio / Natural Frequency  DampingRatio=1  NaturalFrequency=10  SettlingTime=0.59  Overshoot=0  ShowExternalForcePort=off  InitConfig=waypointData_front(1,:)  InitJointVel=0  SimulateUsing=Interpreted execution
  Polynomial Trajectory : robotcorelib/Polynomial Trajectory  WaypointSource=Internal  Waypoints=waypointData_front(1:9,:)'  TimePoints=linspace(15,20,9)  TimeInterval=[ 1, 4 ]  Method=Cubic Polynomial  ParameterSource=Internal  VelocityBoundaryCondition=zeros( 3, 9)  AccelerationBoundaryCondition=zeros( 3, 50)  SimulateUsing=Code generation
  Scope1 : Scope
  Scope2 : Scope
  Terminator : Terminator
  Terminator1 : Terminator
  Output : Outport
  wires:
  Input/1 -> Polynomial Trajectory/1
  Polynomial Trajectory/1 -> Scope1/1, Joint Space Motion Model/1
  Polynomial Trajectory/2 -> Joint Space Motion Model/2
  Joint Space Motion Model/1 -> Scope2/1, Output/1
  Joint Space Motion Model/3 -> Terminator1/1
  Polynomial Trajectory/3 -> Joint Space Motion Model/3
  Joint Space Motion Model/2 -> Terminator/1

== system ele/model/Chassis ==
  ReferenceFrame : sm_lib/Frames and Transforms/Reference Frame
  Visual : sm_lib/Body Elements/Brick Solid  GraphicAmbientColor=[0.15 0.15 0.15 1.0]  BasedOnType=Density  BrickDimensions=[10, 0.5, 10]  BrickDimensionsUnits=m  CenterOfMass=[0, 0, 0]  CenterOfMassUnits=m  GraphicDiffuseColor=[0.5, 0.5, 0.5]  Density=1000  DensityUnits=kg/m^3  DoExposeReferenceFrame=on  GraphicEmissiveColor=[0.0 0.0 0.0 1.0]  ExportEntireGeometry=off  SerializedFrames=<Frames/>  MarkerShape=Sphere  MarkerSize=10  GraphicType=FromGeometry  InertiaType=CalculateFromGeometry  Mass=0  MassUnits=kg  MomentsOfInertia=[0, 0, 0]  MomentsOfInertiaUnits=kg*m^2  GraphicOpacity=1  ProductsOfInertia=[0, 0, 0]  ProductsOfInertiaUnits=kg*m^2  GraphicShininess=75  GraphicSpecularColor=[0.5 0.5 0.5 1.0]  GraphicVisPropType=SimpleVisualProperties
  VisualOriginTransform : sm_lib/Frames and Transforms/Rigid Transform  TranslationMethod=Cartesian  TranslationStandardOffset=0  TranslationStandardOffsetUnits=m  TranslationStandardAxis=+Z  TranslationCartesianOffset=[0, 0, 0]  TranslationCartesianOffsetUnits=m  TranslationROffset=0  TranslationROffsetUnits=m  TranslationZOffset=0  TranslationZOffsetUnits=m  TranslationThetaOffset=0  TranslationThetaOffsetUnits=deg  RotationMethod=RotationSequence  RotationAngleUnits=deg  RotationStandardAxis=+Z  RotationAngle=0.0  RotationArbitraryAxis=[0 0 1]  FollAlignAxisA=+X  BaseAlignAxisA=+Y  FollAlignAxisB=+Y  BaseAlignAxisB=+Z  RotationSequenceAxes=BaseAxes  RotationSequence=XYZ  RotationSequenceAngles=[0, 0, 0]  RotationSequenceAnglesUnits=rad  RotationMatrix=[1 0 0; 0 1 0; 0 0 1]  Quaternion=[1 0 0 0]
  Conn1 : PMIOPort  Side=Right
  Conn2 : PMIOPort  Port=2  Side=Left
  connections:
  Visual/RConn1 -- VisualOriginTransform/RConn1
  Conn2/RConn1 -- VisualOriginTransform/LConn1
  Conn1/RConn1 -- ReferenceFrame/RConn1

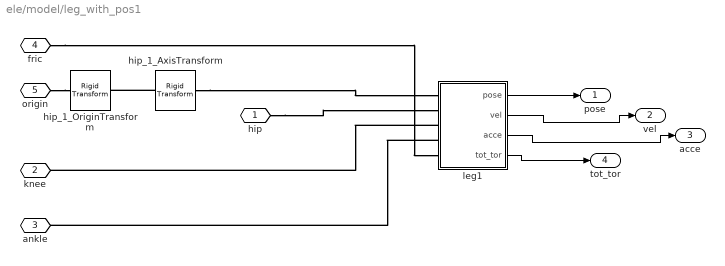
== system ele/model/leg_with_pos1 ==
  hip_1_AxisTransform : sm_lib/Frames and Transforms/Rigid Transform  TranslationMethod=Cartesian  TranslationStandardOffset=0  TranslationStandardOffsetUnits=m  TranslationStandardAxis=+Z  TranslationCartesianOffset=[0, 0, 0]  TranslationCartesianOffsetUnits=m  TranslationROffset=0  TranslationROffsetUnits=m  TranslationZOffset=0  TranslationZOffsetUnits=m  TranslationThetaOffset=0  TranslationThetaOffsetUnits=deg  RotationMethod=ArbitraryAxis  RotationAngleUnits=rad  RotationStandardAxis=+Z  RotationAngle=0  RotationArbitraryAxis=[1, 0, 0]  FollAlignAxisA=+X  BaseAlignAxisA=+Y  FollAlignAxisB=+Y  BaseAlignAxisB=+Z  RotationSequenceAxes=FollowerAxes  RotationSequence=XYX  RotationSequenceAngles=[0 0 0]  RotationSequenceAnglesUnits=deg  RotationMatrix=[1 0 0; 0 1 0; 0 0 1]  Quaternion=[1 0 0 0]
  hip_1_OriginTransform : sm_lib/Frames and Transforms/Rigid Transform  TranslationMethod=Cartesian  TranslationStandardOffset=0  TranslationStandardOffsetUnits=m  TranslationStandardAxis=+Z  TranslationCartesianOffset=[-5, 0, 5]  TranslationCartesianOffsetUnits=m  TranslationROffset=0  TranslationROffsetUnits=m  TranslationZOffset=0  TranslationZOffsetUnits=m  TranslationThetaOffset=0  TranslationThetaOffsetUnits=deg  RotationMethod=RotationSequence  RotationAngleUnits=deg  RotationStandardAxis=+Z  RotationAngle=0.0  RotationArbitraryAxis=[0 0 1]  FollAlignAxisA=+X  BaseAlignAxisA=+Y  FollAlignAxisB=+Y  BaseAlignAxisB=+Z  RotationSequenceAxes=BaseAxes  RotationSequence=XYZ  RotationSequenceAngles=[0, 0, 0]  RotationSequenceAnglesUnits=rad  RotationMatrix=[1 0 0; 0 1 0; 0 0 1]  Quaternion=[1 0 0 0]
  leg1 : Subsystem
  hip : PMIOPort  Side=Left
  knee : PMIOPort  Port=2  Side=Left
  ankle : PMIOPort  Port=3  Side=Left
  fric : PMIOPort  Port=4  Side=Left
  origin : PMIOPort  Port=5  Side=Left
  pose : Outport
  vel : Outport  Port=2
  acce : Outport  Port=3
  tot_tor : Outport  Port=4
  wires:
  leg1/2(vel) -> vel/1
  leg1/4(tot_tor) -> tot_tor/1
  leg1/3(acce) -> acce/1
  leg1/1(pose) -> pose/1
  connections:
  hip_1_AxisTransform/LConn1 -- hip_1_OriginTransform/RConn1
  hip/RConn1 -- leg1/LConn2
  leg1/LConn3 -- knee/RConn1
  hip_1_AxisTransform/RConn1 -- leg1/LConn1
  leg1/LConn4 -- ankle/RConn1
  origin/RConn1 -- hip_1_OriginTransform/LConn1
  fric/RConn1 -- leg1/LConn5

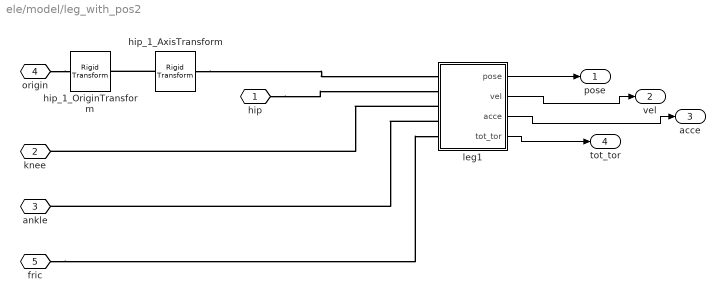
== system ele/model/leg_with_pos2 ==
  hip_1_AxisTransform : sm_lib/Frames and Transforms/Rigid Transform  TranslationMethod=Cartesian  TranslationStandardOffset=0  TranslationStandardOffsetUnits=m  TranslationStandardAxis=+Z  TranslationCartesianOffset=[0, 0, 0]  TranslationCartesianOffsetUnits=m  TranslationROffset=0  TranslationROffsetUnits=m  TranslationZOffset=0  TranslationZOffsetUnits=m  TranslationThetaOffset=0  TranslationThetaOffsetUnits=deg  RotationMethod=ArbitraryAxis  RotationAngleUnits=rad  RotationStandardAxis=+Z  RotationAngle=0  RotationArbitraryAxis=[1, 0, 0]  FollAlignAxisA=+X  BaseAlignAxisA=+Y  FollAlignAxisB=+Y  BaseAlignAxisB=+Z  RotationSequenceAxes=FollowerAxes  RotationSequence=XYX  RotationSequenceAngles=[0 0 0]  RotationSequenceAnglesUnits=deg  RotationMatrix=[1 0 0; 0 1 0; 0 0 1]  Quaternion=[1 0 0 0]
  hip_1_OriginTransform : sm_lib/Frames and Transforms/Rigid Transform  TranslationMethod=Cartesian  TranslationStandardOffset=0  TranslationStandardOffsetUnits=m  TranslationStandardAxis=+Z  TranslationCartesianOffset=[5, 0, 5]  TranslationCartesianOffsetUnits=m  TranslationROffset=0  TranslationROffsetUnits=m  TranslationZOffset=0  TranslationZOffsetUnits=m  TranslationThetaOffset=0  TranslationThetaOffsetUnits=deg  RotationMethod=RotationSequence  RotationAngleUnits=deg  RotationStandardAxis=+Z  RotationAngle=0.0  RotationArbitraryAxis=[0 0 1]  FollAlignAxisA=+X  BaseAlignAxisA=+Y  FollAlignAxisB=+Y  BaseAlignAxisB=+Z  RotationSequenceAxes=BaseAxes  RotationSequence=XYZ  RotationSequenceAngles=[0, 0, 0]  RotationSequenceAnglesUnits=rad  RotationMatrix=[1 0 0; 0 1 0; 0 0 1]  Quaternion=[1 0 0 0]
  leg1 : Subsystem
  hip : PMIOPort  Side=Left
  knee : PMIOPort  Port=2  Side=Left
  ankle : PMIOPort  Port=3  Side=Left
  origin : PMIOPort  Port=4  Side=Left
  fric : PMIOPort  Port=5  Side=Left
  pose : Outport
  vel : Outport  Port=2
  acce : Outport  Port=3
  tot_tor : Outport  Port=4
  wires:
  leg1/1(pose) -> pose/1
  leg1/3(acce) -> acce/1
  leg1/4(tot_tor) -> tot_tor/1
  leg1/2(vel) -> vel/1
  connections:
  origin/RConn1 -- hip_1_OriginTransform/LConn1
  leg1/LConn4 -- ankle/RConn1
  hip_1_AxisTransform/RConn1 -- leg1/LConn1
  leg1/LConn3 -- knee/RConn1
  hip/RConn1 -- leg1/LConn2
  hip_1_AxisTransform/LConn1 -- hip_1_OriginTransform/RConn1
  fric/RConn1 -- leg1/LConn5

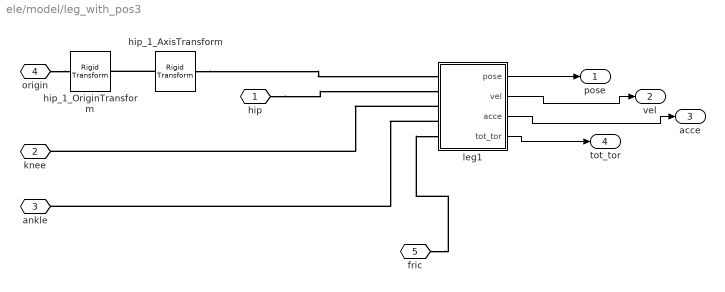
== system ele/model/leg_with_pos3 ==
  hip_1_AxisTransform : sm_lib/Frames and Transforms/Rigid Transform  TranslationMethod=Cartesian  TranslationStandardOffset=0  TranslationStandardOffsetUnits=m  TranslationStandardAxis=+Z  TranslationCartesianOffset=[0, 0, 0]  TranslationCartesianOffsetUnits=m  TranslationROffset=0  TranslationROffsetUnits=m  TranslationZOffset=0  TranslationZOffsetUnits=m  TranslationThetaOffset=0  TranslationThetaOffsetUnits=deg  RotationMethod=ArbitraryAxis  RotationAngleUnits=rad  RotationStandardAxis=+Z  RotationAngle=0  RotationArbitraryAxis=[1, 0, 0]  FollAlignAxisA=+X  BaseAlignAxisA=+Y  FollAlignAxisB=+Y  BaseAlignAxisB=+Z  RotationSequenceAxes=FollowerAxes  RotationSequence=XYX  RotationSequenceAngles=[0 0 0]  RotationSequenceAnglesUnits=deg  RotationMatrix=[1 0 0; 0 1 0; 0 0 1]  Quaternion=[1 0 0 0]
  hip_1_OriginTransform : sm_lib/Frames and Transforms/Rigid Transform  TranslationMethod=Cartesian  TranslationStandardOffset=0  TranslationStandardOffsetUnits=m  TranslationStandardAxis=+Z  TranslationCartesianOffset=[-5, 0, -5]  TranslationCartesianOffsetUnits=m  TranslationROffset=0  TranslationROffsetUnits=m  TranslationZOffset=0  TranslationZOffsetUnits=m  TranslationThetaOffset=0  TranslationThetaOffsetUnits=deg  RotationMethod=RotationSequence  RotationAngleUnits=deg  RotationStandardAxis=+Z  RotationAngle=0.0  RotationArbitraryAxis=[0 0 1]  FollAlignAxisA=+X  BaseAlignAxisA=+Y  FollAlignAxisB=+Y  BaseAlignAxisB=+Z  RotationSequenceAxes=BaseAxes  RotationSequence=XYZ  RotationSequenceAngles=[0, 0, 0]  RotationSequenceAnglesUnits=rad  RotationMatrix=[1 0 0; 0 1 0; 0 0 1]  Quaternion=[1 0 0 0]
  leg1 : Subsystem
  hip : PMIOPort  Side=Left
  knee : PMIOPort  Port=2  Side=Left
  ankle : PMIOPort  Port=3  Side=Left
  origin : PMIOPort  Port=4  Side=Left
  fric : PMIOPort  Port=5  Side=Left
  pose : Outport
  vel : Outport  Port=2
  acce : Outport  Port=3
  tot_tor : Outport  Port=4
  wires:
  leg1/2(vel) -> vel/1
  leg1/4(tot_tor) -> tot_tor/1
  leg1/3(acce) -> acce/1
  leg1/1(pose) -> pose/1
  connections:
  hip_1_AxisTransform/LConn1 -- hip_1_OriginTransform/RConn1
  hip/RConn1 -- leg1/LConn2
  leg1/LConn3 -- knee/RConn1
  hip_1_AxisTransform/RConn1 -- leg1/LConn1
  leg1/LConn4 -- ankle/RConn1
  origin/RConn1 -- hip_1_OriginTransform/LConn1
  fric/RConn1 -- leg1/LConn5

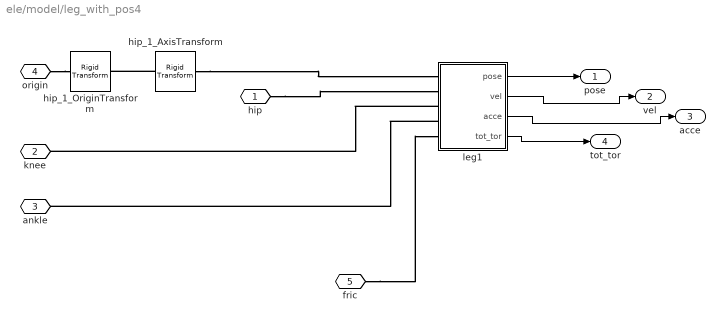
== system ele/model/leg_with_pos4 ==
  hip_1_AxisTransform : sm_lib/Frames and Transforms/Rigid Transform  TranslationMethod=Cartesian  TranslationStandardOffset=0  TranslationStandardOffsetUnits=m  TranslationStandardAxis=+Z  TranslationCartesianOffset=[0, 0, 0]  TranslationCartesianOffsetUnits=m  TranslationROffset=0  TranslationROffsetUnits=m  TranslationZOffset=0  TranslationZOffsetUnits=m  TranslationThetaOffset=0  TranslationThetaOffsetUnits=deg  RotationMethod=ArbitraryAxis  RotationAngleUnits=rad  RotationStandardAxis=+Z  RotationAngle=0  RotationArbitraryAxis=[1, 0, 0]  FollAlignAxisA=+X  BaseAlignAxisA=+Y  FollAlignAxisB=+Y  BaseAlignAxisB=+Z  RotationSequenceAxes=FollowerAxes  RotationSequence=XYX  RotationSequenceAngles=[0 0 0]  RotationSequenceAnglesUnits=deg  RotationMatrix=[1 0 0; 0 1 0; 0 0 1]  Quaternion=[1 0 0 0]
  hip_1_OriginTransform : sm_lib/Frames and Transforms/Rigid Transform  TranslationMethod=Cartesian  TranslationStandardOffset=0  TranslationStandardOffsetUnits=m  TranslationStandardAxis=+Z  TranslationCartesianOffset=[5, 0, -5]  TranslationCartesianOffsetUnits=m  TranslationROffset=0  TranslationROffsetUnits=m  TranslationZOffset=0  TranslationZOffsetUnits=m  TranslationThetaOffset=0  TranslationThetaOffsetUnits=deg  RotationMethod=RotationSequence  RotationAngleUnits=deg  RotationStandardAxis=+Z  RotationAngle=0.0  RotationArbitraryAxis=[0 0 1]  FollAlignAxisA=+X  BaseAlignAxisA=+Y  FollAlignAxisB=+Y  BaseAlignAxisB=+Z  RotationSequenceAxes=BaseAxes  RotationSequence=XYZ  RotationSequenceAngles=[0, 0, 0]  RotationSequenceAnglesUnits=rad  RotationMatrix=[1 0 0; 0 1 0; 0 0 1]  Quaternion=[1 0 0 0]
  leg1 : Subsystem
  hip : PMIOPort  Side=Left
  knee : PMIOPort  Port=2  Side=Left
  ankle : PMIOPort  Port=3  Side=Left
  origin : PMIOPort  Port=4  Side=Left
  fric : PMIOPort  Port=5  Side=Left
  pose : Outport
  vel : Outport  Port=2
  acce : Outport  Port=3
  tot_tor : Outport  Port=4
  wires:
  leg1/1(pose) -> pose/1
  leg1/3(acce) -> acce/1
  leg1/4(tot_tor) -> tot_tor/1
  leg1/2(vel) -> vel/1
  connections:
  origin/RConn1 -- hip_1_OriginTransform/LConn1
  leg1/LConn4 -- ankle/RConn1
  hip_1_AxisTransform/RConn1 -- leg1/LConn1
  leg1/LConn3 -- knee/RConn1
  hip/RConn1 -- leg1/LConn2
  hip_1_AxisTransform/LConn1 -- hip_1_OriginTransform/RConn1
  fric/RConn1 -- leg1/LConn5
